simulink model "SistemaDifusoP7T1ARR"  (R2023a)
settings: Solver=VariableStepAuto  StartTime=0.0  StopTime=60  RelTol=1e-3
libraries: fuzblock x1
settings Model: Creator=flora  LastModifiedBy=Estudiantes
settings OptimizationCC: ReuseModelBlockBuffer=off

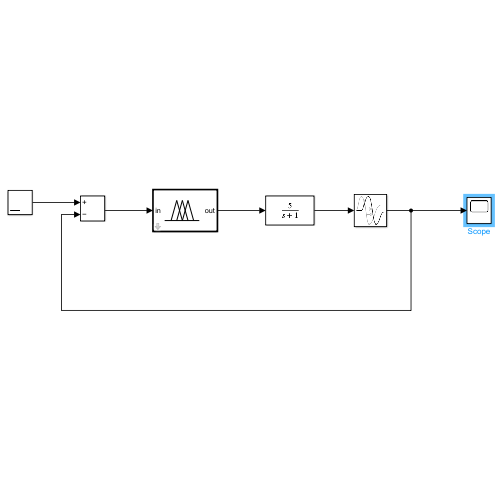
[thumbnail: Simulink's stored preview of the top-level diagram]
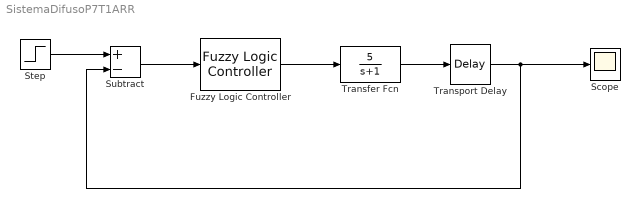
== system SistemaDifusoP7T1ARR ==
  Fuzzy Logic Controller : fuzblock/Fuzzy Logic  Controller  FIS=ControladorDifusoP7T1  OutputSampleNumber=101  DataType=double  FuzzifiedInputs=off  RuleFiringStrengths=off  RuleOutputs=off  AggregatedOutputs=off  SimulateUsing=Interpreted execution  OutOfRangeInputValueMessage=warning  NoRuleFiredMessage=warning  EmptyOutputFuzzySetMessage=warning
  Scope : Scope
  Step : Step  SampleTime=0
  Subtract : Sum  Inputs=+-
  Transfer Fcn : TransferFcn  Numerator=[5]  Denominator=[1 1]
  Transport Delay : TransportDelay  DelayTime=0.2
  wires:
  Transfer Fcn/1 -> Transport Delay/1
  Transport Delay/1 -> Subtract/2, Scope/1
  Step/1 -> Subtract/1
  Subtract/1 -> Fuzzy Logic Controller/1
  Fuzzy Logic Controller/1 -> Transfer Fcn/1
